simulink model "CTC_3PPP"  (R2018b)
settings: Solver=ode3  StartTime=0.0  StopTime=7  FixedStep=1e-3  RelTol=1e-3  EnableMultiTasking=on
undefined symbols (not defined in the file or in its folder): X, Y, Z
libraries: sm_lib x53, nesl_utility x13, simulink x2
(part 1 of 2)
settings Model: Creator=ledan  LastModifiedBy=oattao
settings DataIOCC: LimitDataPoints=on  SaveFormat=Array
settings OptimizationCC: LifeSpan=inf
settings DebuggingCC: UnderspecifiedInitializationDetection=Classic  MergeDetectMultiDrivingBlocksExec=none  SolverPrmCheckMsg=warning  StateNameClashWarn=warning  SFUnexpectedBacktrackingDiag=warning  SFNoUnconditionalDefaultTransitionDiag=warning  SFExecutionAtInitializationDiag=none
settings HardwareCC: ProdBitPerPointer=32  ProdBitPerSizeT=32  ProdBitPerPtrDiffT=32  ProdLargestAtomicFloat=None  ProdIntDivRoundTo=Undefined  ProdEndianess=Unspecified  ProdWordSize=32  ProdHWDeviceType=32-bit Generic
settings ModelReferenceCC: PropagateSignalLabelsOutOfModel=off
settings SFSimCC: SimUseLocalCustomCode=off
settings RTWCC: RTWUseLocalCustomCode=off
settings CodeAppCC: StateflowObjectComments=on
settings GRTTargetCC: TargetLangStandard=C89/C90 (ANSI)  GeneratePreprocessorConditionals=Disable all
settings ConfigComp: CovMetricSettings=dw  CovHtmlReporting=on  CovSaveCumulativeToWorkspaceVar=on  CovSaveSingleToWorkspaceVar=on  CovExternalEMLEnable=off
settings SimscapeCC: SimscapeNormalizeSystem=off
settings ConfigurationSet: Description=SimMechanics 2G

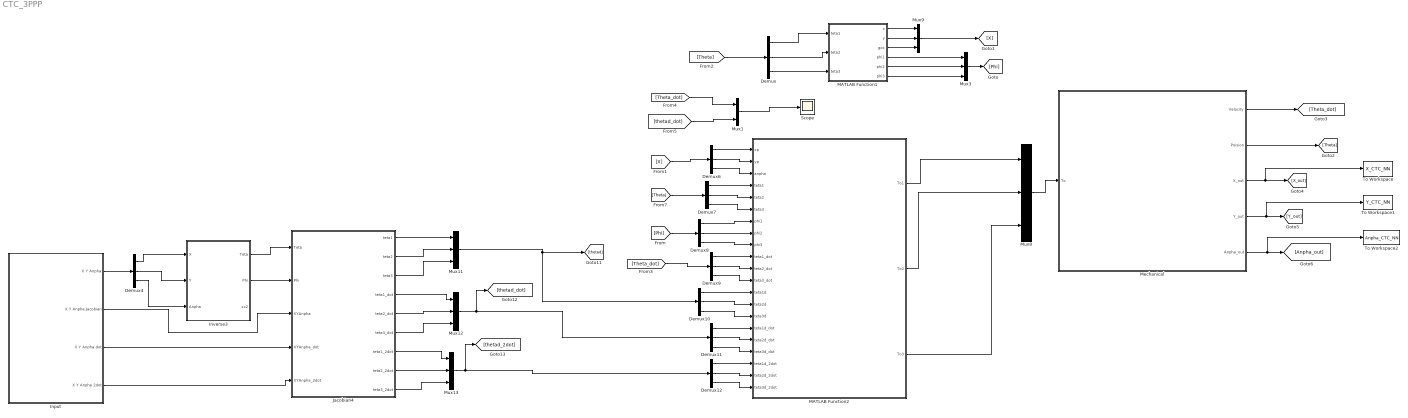
== system CTC_3PPP ==
  Demux{,4,6..12} (9 alike) : Demux  Outputs=3
  Input : Subsystem
  Inverse3 : Subsystem
  Jacobian4 : Subsystem
  MATLAB Function1 : MATLAB Function  TreatAsAtomicUnit=on
  MATLAB Function2 : MATLAB Function  TreatAsAtomicUnit=on
  Mechanical : Subsystem
      mask Display: image('RRR.jpg')
  Mux1 : Mux  Inputs=2
  Mux{3,8..9,11..13} (6 alike) : Mux  Inputs=3
  Scope : Scope
  To Workspace : ToWorkspace  VariableName=X_CTC_NN  SampleTime=-1
  To Workspace1 : ToWorkspace  VariableName=Y_CTC_NN  SampleTime=-1
  To Workspace2 : ToWorkspace  VariableName=Anpha_CTC_NN  SampleTime=-1
  wires:
  Demux/1 -> MATLAB Function1/1(teta1)
  Demux/2 -> MATLAB Function1/2(teta2)
  Demux/3 -> MATLAB Function1/3(teta3)
  MATLAB Function1/4(phi1) -> Mux3/1
  MATLAB Function1/5(phi2) -> Mux3/2
  MATLAB Function1/6(phi3) -> Mux3/3
  Mux12/1 -> [thetad_dot], Demux11/1
  Mux13/1 -> [thetad_2dot], Demux12/1
  Mechanical/1(Velocity) -> [Theta_dot]
  Mechanical/2(Poision) -> [Theta]
  Demux6/1 -> MATLAB Function2/1(xp)
  Demux6/2 -> MATLAB Function2/2(yp)
  Demux6/3 -> MATLAB Function2/3(anpha)
  Demux7/1 -> MATLAB Function2/4(teta1)
  Demux7/2 -> MATLAB Function2/5(teta2)
  Demux7/3 -> MATLAB Function2/6(teta3)
  Demux8/1 -> MATLAB Function2/7(phi1)
  Demux8/2 -> MATLAB Function2/8(phi2)
  Demux8/3 -> MATLAB Function2/9(phi3)
  Demux9/1 -> MATLAB Function2/10(teta1_dot)
  Demux9/2 -> MATLAB Function2/11(teta2_dot)
  Demux9/3 -> MATLAB Function2/12(teta3_dot)
  Demux10/1 -> MATLAB Function2/13(teta1d)
  Demux10/2 -> MATLAB Function2/14(teta2d)
  Demux10/3 -> MATLAB Function2/15(teta3d)
  Demux11/1 -> MATLAB Function2/16(teta1d_dot)
  Demux11/2 -> MATLAB Function2/17(teta2d_dot)
  Demux11/3 -> MATLAB Function2/18(teta3d_dot)
  Demux12/1 -> MATLAB Function2/19(teta1d_2dot)
  Demux12/2 -> MATLAB Function2/20(teta2d_2dot)
  Demux12/3 -> MATLAB Function2/21(teta3d_2dot)
  MATLAB Function1/1(x) -> Mux9/1
  MATLAB Function1/2(y) -> Mux9/2
  MATLAB Function1/3(goc) -> Mux9/3
  Mux3/1 -> [Phi]
  [Phi] -> Demux8/1
  Mux9/1 -> [X]
  [X] -> Demux6/1
  [Theta] -> Demux/1
  [Theta_dot] -> Demux9/1
  [Theta] -> Demux7/1
  Mechanical/3(X_out) -> [X_out], To Workspace/1
  Mechanical/4(Y_out) -> To Workspace1/1, [Y_out]
  Mechanical/5(Anpha_out) -> To Workspace2/1, [Anpha_out]
  Mux11/1 -> [thetad], Demux10/1
  Input/1(X Y Anpha) -> Demux4/1
  Input/2(X Y Anpha Jacobian) -> Jacobian4/3(XYAnpha)
  Input/3(X Y Anpha dot) -> Jacobian4/4(XYAnpha_dot)
  Input/4(X Y Anpha 2dot) -> Jacobian4/5(XYAnpha_2dot)
  Demux4/1 -> Inverse3/1(X)
  Demux4/2 -> Inverse3/2(Y)
  Demux4/3 -> Inverse3/3(Anpha)
  Inverse3/1(Teta) -> Jacobian4/1(Teta)
  Inverse3/2(Phi) -> Jacobian4/2(Phi)
  Jacobian4/1(teta1) -> Mux11/1
  Jacobian4/2(teta2) -> Mux11/2
  Jacobian4/3(teta3) -> Mux11/3
  Jacobian4/4(teta1_dot) -> Mux12/1
  Jacobian4/5(teta2_dot) -> Mux12/2
  Jacobian4/6(teta3_dot) -> Mux12/3
  Jacobian4/7(teta1_2dot) -> Mux13/1
  Jacobian4/8(teta2_2dot) -> Mux13/2
  Jacobian4/9(teta3_2dot) -> Mux13/3
  Mux8/1 -> Mechanical/1(To)
  [Theta_dot] -> Mux1/1
  [thetad_dot] -> Mux1/2
  Mux1/1 -> Scope/1
  MATLAB Function2/1(To1) -> Mux8/1
  MATLAB Function2/2(To2) -> Mux8/2
  MATLAB Function2/3(To3) -> Mux8/3

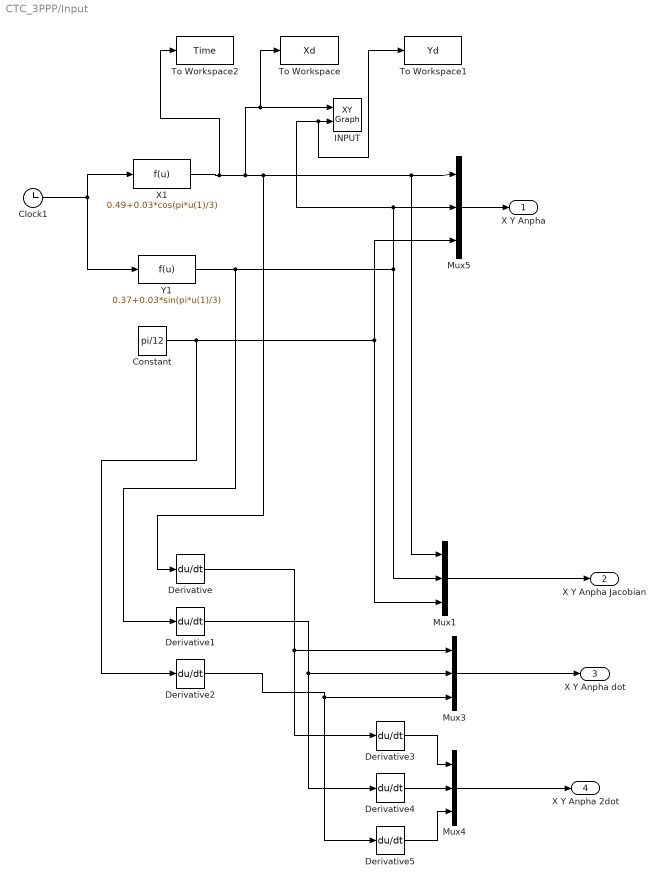
== system CTC_3PPP/Input ==
  Clock1 : Clock
  Constant : Constant  Value=pi/12
  Derivative{,1..5} (6 alike) : Derivative
  INPUT : simulink/Sinks/XY Graph  xmin=0.4  xmax=0.6  ymin=0.3  ymax=0.5  st=-1
  Mux{1,3..5} (4 alike) : Mux  Inputs=3
  To Workspace : ToWorkspace  VariableName=Xd  SampleTime=-1
  To Workspace1 : ToWorkspace  VariableName=Yd  SampleTime=-1
  To Workspace2 : ToWorkspace  VariableName=Time  SaveFormat=Timeseries  SampleTime=-1
  X1 : Fcn  Expr=0.49+0.03*cos(pi*u(1)/3)
  Y1 : Fcn  Expr=0.37+0.03*sin(pi*u(1)/3)
  X Y Anpha : Outport
  X Y Anpha Jacobian : Outport  Port=2
  X Y Anpha dot : Outport  Port=3
  X Y Anpha 2dot : Outport  Port=4
  wires:
  Derivative1/1 -> Mux3/2, Derivative4/1
  Derivative2/1 -> Mux3/3, Derivative5/1
  X1/1 -> To Workspace2/1, Derivative/1, Mux5/1, Mux1/1, To Workspace/1, INPUT/1
  Derivative3/1 -> Mux4/1
  Clock1/1 -> Y1/1, X1/1
  Y1/1 -> Derivative1/1, Mux1/2, To Workspace1/1, INPUT/2, Mux5/2
  Derivative/1 -> Mux3/1, Derivative3/1
  Derivative5/1 -> Mux4/3
  Derivative4/1 -> Mux4/2
  Constant/1 -> Mux1/3, Mux5/3, Derivative2/1
  Mux3/1 -> X Y Anpha dot/1
  Mux4/1 -> X Y Anpha 2dot/1
  Mux1/1 -> X Y Anpha Jacobian/1
  Mux5/1 -> X Y Anpha/1

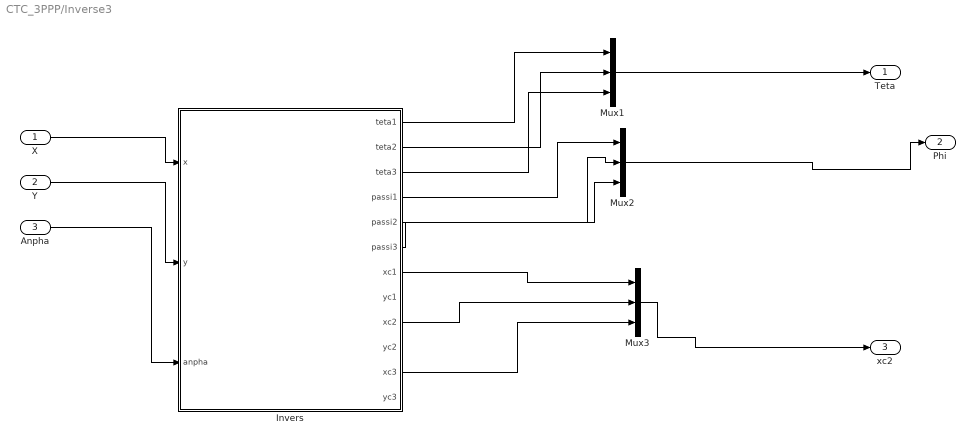
== system CTC_3PPP/Inverse3 ==
  X : Inport
  Y : Inport  Port=2
  Anpha : Inport  Port=3
  Invers : MATLAB Function  TreatAsAtomicUnit=on
  Mux1 : Mux  Inputs=3
  Mux2 : Mux  Inputs=3
  Mux3 : Mux  Inputs=3
  Teta : Outport
  Phi : Outport  Port=2
  xc2 : Outport  Port=3
  wires:
  Mux1/1 -> Teta/1
  Invers/6(passi3) -> Mux2/3
  Invers/3(teta3) -> Mux1/3
  Invers/1(teta1) -> Mux1/1
  Invers/2(teta2) -> Mux1/2
  Invers/4(passi1) -> Mux2/1
  Y/1 -> Invers/2(y)
  Anpha/1 -> Invers/3(anpha)
  X/1 -> Invers/1(x)
  Mux2/1 -> Phi/1
  Invers/5(passi2) -> Mux2/2
  Invers/7(xc1) -> Mux3/1
  Invers/11(xc3) -> Mux3/3
  Mux3/1 -> xc2/1
  Invers/9(xc2) -> Mux3/2

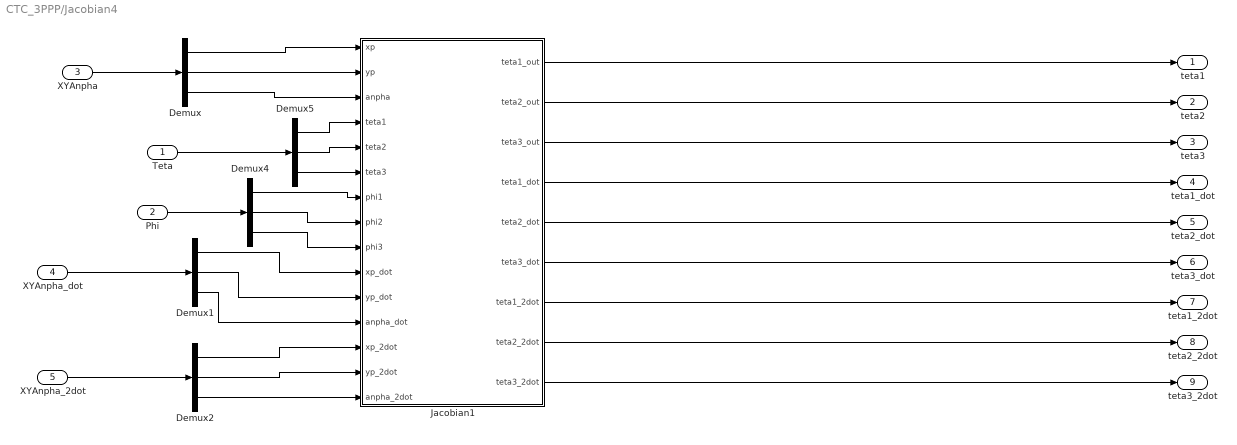
== system CTC_3PPP/Jacobian4 ==
  Teta : Inport
  Phi : Inport  Port=2
  XYAnpha : Inport  Port=3
  XYAnpha_dot : Inport  Port=4
  XYAnpha_2dot : Inport  Port=5
  Demux{,1..2,4..5} (5 alike) : Demux  Outputs=3
  Jacobian1 : MATLAB Function  TreatAsAtomicUnit=on
  teta1 : Outport
  teta2 : Outport  Port=2
  teta3 : Outport  Port=3
  teta1_dot : Outport  Port=4
  teta2_dot : Outport  Port=5
  teta3_dot : Outport  Port=6
  teta1_2dot : Outport  Port=7
  teta2_2dot : Outport  Port=8
  teta3_2dot : Outport  Port=9
  wires:
  XYAnpha_2dot/1 -> Demux2/1
  XYAnpha_dot/1 -> Demux1/1
  XYAnpha/1 -> Demux/1
  Demux/1 -> Jacobian1/1(xp)
  Demux4/2 -> Jacobian1/8(phi2)
  Demux2/3 -> Jacobian1/15(anpha_2dot)
  Demux2/1 -> Jacobian1/13(xp_2dot)
  Demux5/2 -> Jacobian1/5(teta2)
  Demux1/1 -> Jacobian1/10(xp_dot)
  Demux5/1 -> Jacobian1/4(teta1)
  Demux/2 -> Jacobian1/2(yp)
  Demux1/2 -> Jacobian1/11(yp_dot)
  Demux1/3 -> Jacobian1/12(anpha_dot)
  Demux2/2 -> Jacobian1/14(yp_2dot)
  Jacobian1/1(teta1_out) -> teta1/1
  Phi/1 -> Demux4/1
  Demux4/1 -> Jacobian1/7(phi1)
  Demux/3 -> Jacobian1/3(anpha)
  Demux5/3 -> Jacobian1/6(teta3)
  Teta/1 -> Demux5/1
  Jacobian1/3(teta3_out) -> teta3/1
  Demux4/3 -> Jacobian1/9(phi3)
  Jacobian1/2(teta2_out) -> teta2/1
  Jacobian1/6(teta3_dot) -> teta3_dot/1
  Jacobian1/4(teta1_dot) -> teta1_dot/1
  Jacobian1/5(teta2_dot) -> teta2_dot/1
  Jacobian1/7(teta1_2dot) -> teta1_2dot/1
  Jacobian1/8(teta2_2dot) -> teta2_2dot/1
  Jacobian1/9(teta3_2dot) -> teta3_2dot/1

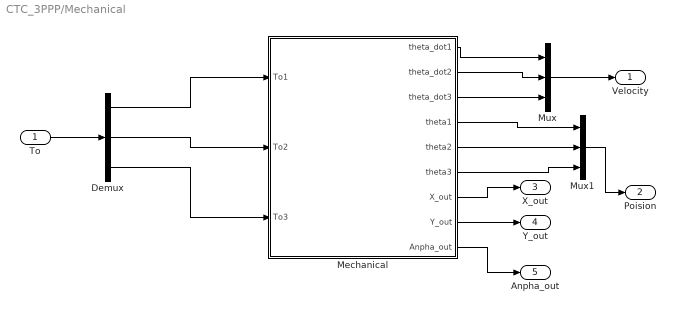
== system CTC_3PPP/Mechanical ==
  To : Inport
  Demux : Demux  Outputs=3
  Mechanical : Subsystem
  Mux : Mux  Inputs=3
  Mux1 : Mux  Inputs=3
  Velocity : Outport
  Poision : Outport  Port=2
  X_out : Outport  Port=3
  Y_out : Outport  Port=4
  Anpha_out : Outport  Port=5
  wires:
  Mechanical/3(theta_dot3) -> Mux/3
  Mechanical/1(theta_dot1) -> Mux/1
  Mechanical/5(theta2) -> Mux1/2
  Mechanical/6(theta3) -> Mux1/3
  Mechanical/4(theta1) -> Mux1/1
  Mux1/1 -> Poision/1
  Mechanical/2(theta_dot2) -> Mux/2
  To/1 -> Demux/1
  Mux/1 -> Velocity/1
  Demux/2 -> Mechanical/2(To2)
  Demux/3 -> Mechanical/3(To3)
  Mechanical/7(X_out) -> X_out/1
  Mechanical/8(Y_out) -> Y_out/1
  Mechanical/9(Anpha_out) -> Anpha_out/1
  Demux/1 -> Mechanical/1(To1)

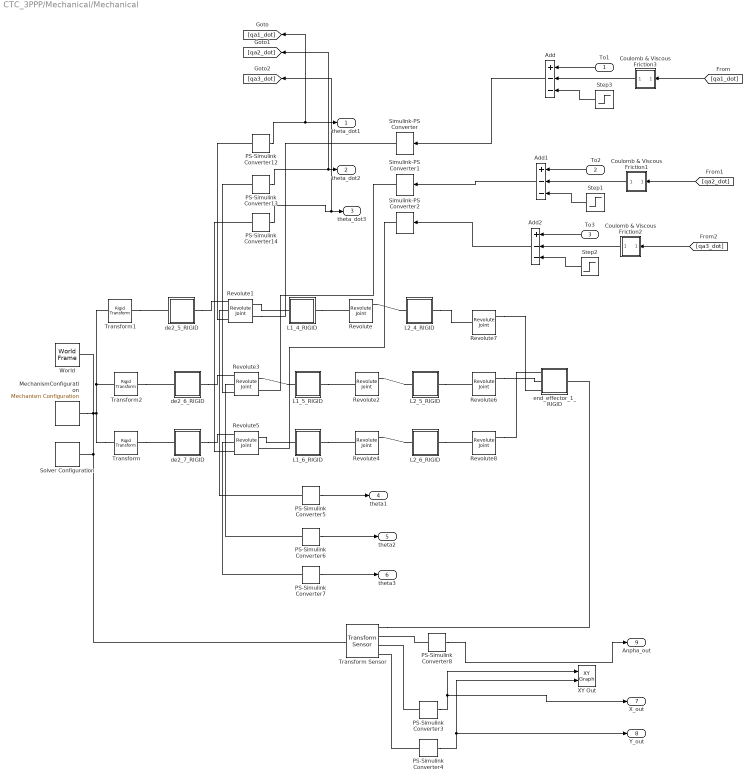
== system CTC_3PPP/Mechanical/Mechanical ==
  To1 : Inport
  To2 : Inport  Port=2
  To3 : Inport  Port=3
  Add : Sum  Inputs=+--
  Add1 : Sum  Inputs=+--
  Add2 : Sum  Inputs=+--
  Coulomb & Viscous Friction1 : Subsystem  AncestorBlock=simulink/Discontinuities/Coulomb & Viscous Friction  mask(Coulombic and Viscous Friction){offset=0.4, gain=0.5}
      mask prompts: offset "Coulomb friction value (Offset):"; gain "Coefficient of viscous friction (Gain):"
      mask help:
      | A discontinuity offset at zero models coulomb friction.  Linear gain models viscous friction.
      | y = sign(x) * (Gain * abs(x) + Offset)
      mask init:
      | dblOffset = double(offset(1));
      | dblGain = double(gain(1));
      | x=max(dblOffset,dblGain+dblOffset);
      mask Help:
      | This block has a discontinuity
      | at zero and a linear gain afterward.
      | y= sign(x)*(Gain*abs(x)+Offset)
      mask Display:
      | plot([-1 0 0 1],[-dblGain-dblOffset, -dblOffset, ...
      |     dblOffset, dblGain+dblOffset],...
      |     [-1 1],[0 0],[0 0],[-x,x])
  Coulomb & Viscous Friction2 : Subsystem  AncestorBlock=simulink/Discontinuities/Coulomb & Viscous Friction  mask(Coulombic and Viscous Friction){offset=0.4, gain=0.5}
      mask prompts: offset "Coulomb friction value (Offset):"; gain "Coefficient of viscous friction (Gain):"
      mask help:
      | A discontinuity offset at zero models coulomb friction.  Linear gain models viscous friction.
      | y = sign(x) * (Gain * abs(x) + Offset)
      mask init:
      | dblOffset = double(offset(1));
      | dblGain = double(gain(1));
      | x=max(dblOffset,dblGain+dblOffset);
      mask Help:
      | This block has a discontinuity
      | at zero and a linear gain afterward.
      | y= sign(x)*(Gain*abs(x)+Offset)
      mask Display:
      | plot([-1 0 0 1],[-dblGain-dblOffset, -dblOffset, ...
      |     dblOffset, dblGain+dblOffset],...
      |     [-1 1],[0 0],[0 0],[-x,x])
  Coulomb & Viscous Friction3 : Subsystem  AncestorBlock=simulink/Discontinuities/Coulomb & Viscous Friction  mask(Coulombic and Viscous Friction){offset=0.4, gain=0.5}
      mask prompts: offset "Coulomb friction value (Offset):"; gain "Coefficient of viscous friction (Gain):"
      mask help:
      | A discontinuity offset at zero models coulomb friction.  Linear gain models viscous friction.
      | y = sign(x) * (Gain * abs(x) + Offset)
      mask init:
      | dblOffset = double(offset(1));
      | dblGain = double(gain(1));
      | x=max(dblOffset,dblGain+dblOffset);
      mask Help:
      | This block has a discontinuity
      | at zero and a linear gain afterward.
      | y= sign(x)*(Gain*abs(x)+Offset)
      mask Display:
      | plot([-1 0 0 1],[-dblGain-dblOffset, -dblOffset, ...
      |     dblOffset, dblGain+dblOffset],...
      |     [-1 1],[0 0],[0 0],[-x,x])
  L1_4_RIGID : Subsystem
  L1_5_RIGID : Subsystem
  L1_6_RIGID : Subsystem
  L2_4_RIGID : Subsystem
  L2_5_RIGID : Subsystem
  L2_6_RIGID : Subsystem
  MechanismConfiguration : sm_lib/Utilities/Mechanism Configuration  UniformGravity=Constant  GravityVector=[0 -9.81 0]  GravityUnits=m/s^2  LinearizationDelta=0.001
  PS-Simulink Converter{3..8,12..14} (9 alike) : nesl_utility/PS-Simulink Converter  PhysicalDomain=network_engine_domain  SubClassName=ps_output  LeftPortType=input  RightPortType=output  PseudoPeriodic=off  Frequencies=[]  Unit=1  AffineConversion=off
  Revolute : sm_lib/Joints/Revolute Joint  SenseConstraintForce=off  SenseConstraintForceX=off  SenseConstraintForceY=off  SenseConstraintForceZ=off  SenseConstraintTorque=off  SenseConstraintTorqueX=off  SenseConstraintTorqueY=off  SenseConstraintTorqueZ=off  SenseTotalForce=off  SenseTotalForceX=off  SenseTotalForceY=off  SenseTotalForceZ=off  SenseTotalTorque=off  SenseTotalTorqueX=off  SenseTotalTorqueY=off  SenseTotalTorqueZ=off  CompositeWrenchDir=FollowerOnBase  CompositeWrenchFrame=BaseFrame  EquilibriumPosition=0  EquilibriumPositionUnits=rad  SpringStiffness=0  SpringStiffnessUnits=m*N/rad  DampingCoefficient=0  DampingCoefficientUnits=m*s*N/rad  TorqueActuationMode=NoTorque  MotionActuationMode=ComputedMotion  SensePosition=on  SenseVelocity=off  SenseAcceleration=off  SenseTorqueForce=off  PositionTargetSpecify=on  PositionTargetPriority=Low  PositionTargetValue=-2.4388  PositionTargetValueUnits=rad  VelocityTargetSpecify=off  VelocityTargetPriority=High  VelocityTargetValue=0  VelocityTargetValueUnits=deg/s
  Revolute1 : sm_lib/Joints/Revolute Joint  SenseConstraintForce=off  SenseConstraintForceX=off  SenseConstraintForceY=off  SenseConstraintForceZ=off  SenseConstraintTorque=off  SenseConstraintTorqueX=off  SenseConstraintTorqueY=off  SenseConstraintTorqueZ=off  SenseTotalForce=off  SenseTotalForceX=off  SenseTotalForceY=off  SenseTotalForceZ=off  SenseTotalTorque=off  SenseTotalTorqueX=off  SenseTotalTorqueY=off  SenseTotalTorqueZ=off  CompositeWrenchDir=FollowerOnBase  CompositeWrenchFrame=BaseFrame  EquilibriumPosition=0  EquilibriumPositionUnits=rad  SpringStiffness=0  SpringStiffnessUnits=m*N/rad  DampingCoefficient=0  DampingCoefficientUnits=m*s*N/rad  TorqueActuationMode=InputTorque  MotionActuationMode=ComputedMotion  SensePosition=on  SenseVelocity=on  SenseAcceleration=off  SenseTorqueForce=off  PositionTargetSpecify=on  PositionTargetPriority=Low  PositionTargetValue=2.1636  PositionTargetValueUnits=rad  VelocityTargetSpecify=off  VelocityTargetPriority=High  VelocityTargetValue=0  VelocityTargetValueUnits=deg/s
  Revolute2 : sm_lib/Joints/Revolute Joint  SenseConstraintForce=off  SenseConstraintForceX=off  SenseConstraintForceY=off  SenseConstraintForceZ=off  SenseConstraintTorque=off  SenseConstraintTorqueX=off  SenseConstraintTorqueY=off  SenseConstraintTorqueZ=off  SenseTotalForce=off  SenseTotalForceX=off  SenseTotalForceY=off  SenseTotalForceZ=off  SenseTotalTorque=off  SenseTotalTorqueX=off  SenseTotalTorqueY=off  SenseTotalTorqueZ=off  CompositeWrenchDir=FollowerOnBase  CompositeWrenchFrame=BaseFrame  EquilibriumPosition=0  EquilibriumPositionUnits=rad  SpringStiffness=0  SpringStiffnessUnits=m*N/rad  DampingCoefficient=0  DampingCoefficientUnits=m*s*N/rad  TorqueActuationMode=NoTorque  MotionActuationMode=ComputedMotion  SensePosition=on  SenseVelocity=off  SenseAcceleration=off  SenseTorqueForce=off  PositionTargetSpecify=off  PositionTargetPriority=Low  PositionTargetValue=-2.1897  PositionTargetValueUnits=rad  VelocityTargetSpecify=off  VelocityTargetPriority=High  VelocityTargetValue=0  VelocityTargetValueUnits=deg/s
  Revolute3 : sm_lib/Joints/Revolute Joint  SenseConstraintForce=off  SenseConstraintForceX=off  SenseConstraintForceY=off  SenseConstraintForceZ=off  SenseConstraintTorque=off  SenseConstraintTorqueX=off  SenseConstraintTorqueY=off  SenseConstraintTorqueZ=off  SenseTotalForce=off  SenseTotalForceX=off  SenseTotalForceY=off  SenseTotalForceZ=off  SenseTotalTorque=off  SenseTotalTorqueX=off  SenseTotalTorqueY=off  SenseTotalTorqueZ=off  CompositeWrenchDir=FollowerOnBase  CompositeWrenchFrame=BaseFrame  EquilibriumPosition=0  EquilibriumPositionUnits=rad  SpringStiffness=0  SpringStiffnessUnits=m*N/rad  DampingCoefficient=0  DampingCoefficientUnits=m*s*N/rad  TorqueActuationMode=InputTorque  MotionActuationMode=ComputedMotion  SensePosition=on  SenseVelocity=on  SenseAcceleration=off  SenseTorqueForce=off  PositionTargetSpecify=on  PositionTargetPriority=Low  PositionTargetValue=4.02  PositionTargetValueUnits=rad  VelocityTargetSpecify=off  VelocityTargetPriority=High  VelocityTargetValue=0  VelocityTargetValueUnits=deg/s
  Revolute4 : sm_lib/Joints/Revolute Joint  SenseConstraintForce=off  SenseConstraintForceX=off  SenseConstraintForceY=off  SenseConstraintForceZ=off  SenseConstraintTorque=off  SenseConstraintTorqueX=off  SenseConstraintTorqueY=off  SenseConstraintTorqueZ=off  SenseTotalForce=off  SenseTotalForceX=off  SenseTotalForceY=off  SenseTotalForceZ=off  SenseTotalTorque=off  SenseTotalTorqueX=off  SenseTotalTorqueY=off  SenseTotalTorqueZ=off  CompositeWrenchDir=FollowerOnBase  CompositeWrenchFrame=BaseFrame  EquilibriumPosition=0  EquilibriumPositionUnits=rad  SpringStiffness=0  SpringStiffnessUnits=m*N/rad  DampingCoefficient=0  DampingCoefficientUnits=m*s*N/rad  TorqueActuationMode=NoTorque  MotionActuationMode=ComputedMotion  SensePosition=on  SenseVelocity=off  SenseAcceleration=off  SenseTorqueForce=off  PositionTargetSpecify=off  PositionTargetPriority=Low  PositionTargetValue=2.7158  PositionTargetValueUnits=rad  VelocityTargetSpecify=off  VelocityTargetPriority=High  VelocityTargetValue=0  VelocityTargetValueUnits=deg/s
  Revolute5 : sm_lib/Joints/Revolute Joint  SenseConstraintForce=off  SenseConstraintForceX=off  SenseConstraintForceY=off  SenseConstraintForceZ=off  SenseConstraintTorque=off  SenseConstraintTorqueX=off  SenseConstraintTorqueY=off  SenseConstraintTorqueZ=off  SenseTotalForce=off  SenseTotalForceX=off  SenseTotalForceY=off  SenseTotalForceZ=off  SenseTotalTorque=off  SenseTotalTorqueX=off  SenseTotalTorqueY=off  SenseTotalTorqueZ=off  CompositeWrenchDir=FollowerOnBase  CompositeWrenchFrame=BaseFrame  EquilibriumPosition=0  EquilibriumPositionUnits=rad  SpringStiffness=0  SpringStiffnessUnits=m*N/rad  DampingCoefficient=0  DampingCoefficientUnits=m*s*N/rad  TorqueActuationMode=InputTorque  MotionActuationMode=ComputedMotion  SensePosition=on  SenseVelocity=on  SenseAcceleration=off  SenseTorqueForce=off  PositionTargetSpecify=on  PositionTargetPriority=Low  PositionTargetValue=0.5  PositionTargetValueUnits=rad  VelocityTargetSpecify=off  VelocityTargetPriority=High  VelocityTargetValue=0  VelocityTargetValueUnits=deg/s
  Revolute6 : sm_lib/Joints/Revolute Joint  SenseConstraintForce=off  SenseConstraintForceX=off  SenseConstraintForceY=off  SenseConstraintForceZ=off  SenseConstraintTorque=off  SenseConstraintTorqueX=off  SenseConstraintTorqueY=off  SenseConstraintTorqueZ=off  SenseTotalForce=off  SenseTotalForceX=off  SenseTotalForceY=off  SenseTotalForceZ=off  SenseTotalTorque=off  SenseTotalTorqueX=off  SenseTotalTorqueY=off  SenseTotalTorqueZ=off  CompositeWrenchDir=FollowerOnBase  CompositeWrenchFrame=BaseFrame  EquilibriumPosition=0  EquilibriumPositionUnits=rad  SpringStiffness=0  SpringStiffnessUnits=m*N/rad  DampingCoefficient=0  DampingCoefficientUnits=m*s*N/rad  TorqueActuationMode=NoTorque  MotionActuationMode=ComputedMotion  SensePosition=on  SenseVelocity=off  SenseAcceleration=off  SenseTorqueForce=off  PositionTargetSpecify=off  PositionTargetPriority=Low  PositionTargetValue=0  PositionTargetValueUnits=rad  VelocityTargetSpecify=off  VelocityTargetPriority=High  VelocityTargetValue=0  VelocityTargetValueUnits=deg/s
  Revolute7 : sm_lib/Joints/Revolute Joint  SenseConstraintForce=off  SenseConstraintForceX=off  SenseConstraintForceY=off  SenseConstraintForceZ=off  SenseConstraintTorque=off  SenseConstraintTorqueX=off  SenseConstraintTorqueY=off  SenseConstraintTorqueZ=off  SenseTotalForce=off  SenseTotalForceX=off  SenseTotalForceY=off  SenseTotalForceZ=off  SenseTotalTorque=off  SenseTotalTorqueX=off  SenseTotalTorqueY=off  SenseTotalTorqueZ=off  CompositeWrenchDir=FollowerOnBase  CompositeWrenchFrame=BaseFrame  EquilibriumPosition=0  EquilibriumPositionUnits=rad  SpringStiffness=0  SpringStiffnessUnits=m*N/rad  DampingCoefficient=0  DampingCoefficientUnits=m*s*N/rad  TorqueActuationMode=NoTorque  MotionActuationMode=ComputedMotion  SensePosition=on  SenseVelocity=off  SenseAcceleration=off  SenseTorqueForce=off  PositionTargetSpecify=off  PositionTargetPriority=Low  PositionTargetValue=0  PositionTargetValueUnits=rad  VelocityTargetSpecify=off  VelocityTargetPriority=High  VelocityTargetValue=0  VelocityTargetValueUnits=deg/s
  Revolute8 : sm_lib/Joints/Revolute Joint  SenseConstraintForce=off  SenseConstraintForceX=off  SenseConstraintForceY=off  SenseConstraintForceZ=off  SenseConstraintTorque=off  SenseConstraintTorqueX=off  SenseConstraintTorqueY=off  SenseConstraintTorqueZ=off  SenseTotalForce=off  SenseTotalForceX=off  SenseTotalForceY=off  SenseTotalForceZ=off  SenseTotalTorque=off  SenseTotalTorqueX=off  SenseTotalTorqueY=off  SenseTotalTorqueZ=off  CompositeWrenchDir=FollowerOnBase  CompositeWrenchFrame=BaseFrame  EquilibriumPosition=0  EquilibriumPositionUnits=rad  SpringStiffness=0  SpringStiffnessUnits=m*N/rad  DampingCoefficient=0  DampingCoefficientUnits=m*s*N/rad  TorqueActuationMode=NoTorque  MotionActuationMode=ComputedMotion  SensePosition=on  SenseVelocity=off  SenseAcceleration=off  SenseTorqueForce=off  PositionTargetSpecify=off  PositionTargetPriority=Low  PositionTargetValue=0  PositionTargetValueUnits=rad  VelocityTargetSpecify=off  VelocityTargetPriority=High  VelocityTargetValue=0  VelocityTargetValueUnits=deg/s
  Simulink-PS Converter : nesl_utility/Simulink-PS Converter  PhysicalDomain=network_engine_domain  SubClassName=ps_input  LeftPortType=input  RightPortType=output  PseudoPeriodic=off  Frequencies=[]  NoiseDistribution=none  NoiseParameters=[]  Unit=1  AffineConversion=off  FilteringAndDerivatives=zero  SimscapeFilterOrder=1  InputFilterTimeConstant=0.001  UdotUserProvided=1
  Simulink-PS Converter1 : nesl_utility/Simulink-PS Converter  PhysicalDomain=network_engine_domain  SubClassName=ps_input  LeftPortType=input  RightPortType=output  PseudoPeriodic=off  Frequencies=[]  NoiseDistribution=none  NoiseParameters=[]  Unit=1  AffineConversion=off  FilteringAndDerivatives=zero  SimscapeFilterOrder=1  InputFilterTimeConstant=0.001  UdotUserProvided=1
  Simulink-PS Converter2 : nesl_utility/Simulink-PS Converter  PhysicalDomain=network_engine_domain  SubClassName=ps_input  LeftPortType=input  RightPortType=output  PseudoPeriodic=off  Frequencies=[]  NoiseDistribution=none  NoiseParameters=[]  Unit=1  AffineConversion=off  FilteringAndDerivatives=zero  SimscapeFilterOrder=1  InputFilterTimeConstant=0.001  UdotUserProvided=1
  Solver Configuration : nesl_utility/Solver Configuration  PhysicalDomain=network_engine_domain  SubClassName=solver  LeftPortType=input  RightPortType=generic  Tones=[]  Harmonics=[]  SimulateNoise=off  Profile=off  UseLocalSampling=off  EnableSwitchedLinearOptims=on  FrequencyDomain=off  UseCCode=off  RelTol=0.001  AbsTol=1e-06  MinStep=1e-09  ToWorkspace=off  RevertToSquareIcSolve=off  NumHomotopyIterations=100  PhasorMode=off  PhasorModeNumHarmonics=1  DoDC=off  ResidualTolerance=1e-09  UseLocalSolver=off  LocalSolverChoice=NE_BACKWARD_EULER_ADVANCER  LocalSolverSampleTime=0.001  DoFixedCost=off  MaxNonlinIter=3  MaxModeIter=2  LinearAlgebra=Sparse  EquationFormulation=NE_TIME_EF  DelaysMemoryBudget=1024  AutomaticFiltering=on  FilteringTimeConstant=0.001  PartitionStorageMethod=AS_NEEDED  PartitionMemoryBudget=1024
  Step1 : Step  Time=0.5  After=0.001  SampleTime=0
  Step2 : Step  Time=0.5  After=0.001  SampleTime=0
  Step3 : Step  Time=0.5  After=0.001  SampleTime=0
  Transform : sm_lib/Frames and Transforms/Rigid Transform  TranslationMethod=Cartesian  TranslationStandardOffset=0  TranslationLengthUnit=mm  TranslationStandardAxis=+Z  TranslationCartesianOffset=[500 0 866.02500000000009]  TranslationROffset=0  TranslationROffsetUnits=m  TranslationZOffset=0  TranslationZOffsetUnits=m  TranslationThetaOffset=0  TranslationThetaOffsetUnits=deg  RotationMethod=None  RotationAngleUnits=deg  RotationStandardAxis=+Z  RotationAngle=0  RotationArbitraryAxis=[0 0 1]  FollAlignAxisA=+X  BaseAlignAxisA=+Y  FollAlignAxisB=+Y  BaseAlignAxisB=+Z  RotationSequenceAxes=FollowerAxes  RotationSequence=XYX  RotationSequenceAngles=[0 0 0]  RotationSequenceAnglesUnits=deg  RotationMatrix=[1 0 0; 0 1 0; 0 0 1]
  Transform Sensor : sm_lib/Frames and Transforms/Transform Sensor  MeasurementFrame=World  SenseAngle=on  SenseAxis=off  SenseAngle1=off  SenseAngle2=off  SenseAngle3=off  SenseQ=off  SenseR=off  SenseOmegaX=off  SenseOmegaY=off  SenseOmegaZ=off  SenseOmega1=off  SenseOmega2=off  SenseOmega3=off  SenseQDot=off  SenseRDot=off  SenseAlphaX=off  SenseAlphaY=off  SenseAlphaZ=off  SenseAlpha1=off  SenseAlpha2=off  SenseAlpha3=off  SenseQDDot=off  SenseRDDot=off  SenseX=on  SenseY=off  SenseZ=on  SenseRad=off  SenseAzim=off  SenseDist=off  SenseInc=off  SenseXDot=off  SenseYDot=off  SenseZDot=off  SenseRadDot=off  SenseAzimDot=off  SenseDistDot=off  SenseIncDot=off  SenseXDDot=off  SenseYDDot=off  SenseZDDot=off  SenseRadDDot=off  SenseAzimDDot=off  SenseDistDDot=off  SenseIncDDot=off
  Transform1 : sm_lib/Frames and Transforms/Rigid Transform  TranslationMethod=None  TranslationStandardOffset=0  TranslationLengthUnit=m  TranslationStandardAxis=+Z  TranslationCartesianOffset=[0 0 0]  TranslationROffset=0  TranslationROffsetUnits=m  TranslationZOffset=0  TranslationZOffsetUnits=m  TranslationThetaOffset=0  TranslationThetaOffsetUnits=deg  RotationMethod=None  RotationAngleUnits=deg  RotationStandardAxis=+Z  RotationAngle=0  RotationArbitraryAxis=[0 0 1]  FollAlignAxisA=+X  BaseAlignAxisA=+Y  FollAlignAxisB=+Y  BaseAlignAxisB=+Z  RotationSequenceAxes=FollowerAxes  RotationSequence=XYX  RotationSequenceAngles=[0 0 0]  RotationSequenceAnglesUnits=deg  RotationMatrix=[1 0 0; 0 1 0; 0 0 1]
  Transform2 : sm_lib/Frames and Transforms/Rigid Transform  TranslationMethod=Cartesian  TranslationStandardOffset=0  TranslationLengthUnit=mm  TranslationStandardAxis=+Z  TranslationCartesianOffset=[1000 0 0]  TranslationROffset=0  TranslationROffsetUnits=m  TranslationZOffset=0  TranslationZOffsetUnits=m  TranslationThetaOffset=0  TranslationThetaOffsetUnits=deg  RotationMethod=None  RotationAngleUnits=deg  RotationStandardAxis=+Z  RotationAngle=0  RotationArbitraryAxis=[0 0 1]  FollAlignAxisA=+X  BaseAlignAxisA=+Y  FollAlignAxisB=+Y  BaseAlignAxisB=+Z  RotationSequenceAxes=FollowerAxes  RotationSequence=XYX  RotationSequenceAngles=[0 0 0]  RotationSequenceAnglesUnits=deg  RotationMatrix=[1 0 0; 0 1 0; 0 0 1]
  World : sm_lib/Frames and Transforms/World Frame
  XY Out : simulink/Sinks/XY Graph  xmin=0.4  xmax=0.6  ymin=0.3  ymax=0.5  st=-1
  de2_5_RIGID : Subsystem
  de2_6_RIGID : Subsystem
  de2_7_RIGID : Subsystem
  end_effector_1_RIGID : Subsystem
  theta_dot1 : Outport
  theta_dot2 : Outport  Port=2
  theta_dot3 : Outport  Port=3
  theta1 : Outport  Port=4
  theta2 : Outport  Port=5
  theta3 : Outport  Port=6
  X_out : Outport  Port=7
  Y_out : Outport  Port=8
  Anpha_out : Outport  Port=9
  wires:
  PS-Simulink Converter8/1 -> Anpha_out/1
  Add1/1 -> Simulink-PS Converter1/1
  Add/1 -> Simulink-PS Converter/1
  Add2/1 -> Simulink-PS Converter2/1
  PS-Simulink Converter3/1 -> X_out/1, XY Out/1
  PS-Simulink Converter4/1 -> Y_out/1, XY Out/2
  PS-Simulink Converter5/1 -> theta1/1
  PS-Simulink Converter7/1 -> theta3/1
  PS-Simulink Converter6/1 -> theta2/1
  PS-Simulink Converter14/1 -> [qa3_dot], theta_dot3/1
  PS-Simulink Converter13/1 -> [qa2_dot], theta_dot2/1
  Coulomb & Viscous Friction3/1(Out1) -> Add/2
  Step3/1 -> Add/3
  [qa1_dot] -> Coulomb & Viscous Friction3/1(In1)
  To1/1 -> Add/1
  PS-Simulink Converter12/1 -> [qa1_dot], theta_dot1/1
  Coulomb & Viscous Friction1/1(Out1) -> Add1/2
  Step1/1 -> Add1/3
  [qa2_dot] -> Coulomb & Viscous Friction1/1(In1)
  To2/1 -> Add1/1
  Coulomb & Viscous Friction2/1(Out1) -> Add2/2
  Step2/1 -> Add2/3
  [qa3_dot] -> Coulomb & Viscous Friction2/1(In1)
  To3/1 -> Add2/1
  connections:
  de2_6_RIGID/RConn1 -- Revolute3/RConn1
  PS-Simulink Converter3/LConn1 -- Transform Sensor/RConn3
  Revolute5/LConn1 -- L1_6_RIGID/LConn1
  de2_7_RIGID/RConn1 -- Revolute5/RConn1
  L2_4_RIGID/RConn1 -- Revolute7/LConn1
  PS-Simulink Converter4/LConn1 -- Transform Sensor/RConn4
  PS-Simulink Converter8/LConn1 -- Transform Sensor/RConn2
  Simulink-PS Converter1/RConn1 -- Revolute3/LConn2
  Revolute1/LConn2 -- Simulink-PS Converter/RConn1
  L2_5_RIGID/RConn1 -- Revolute6/LConn1
  Simulink-PS Converter2/RConn1 -- Revolute5/LConn2
  Transform/LConn1 -- Transform1/LConn1 -- Transform2/LConn1 -- MechanismConfiguration/RConn1 -- Transform Sensor/LConn1 -- Solver Configuration/RConn1 -- World/RConn1
  L1_4_RIGID/RConn1 -- Revolute/LConn1
  L2_6_RIGID/LConn1 -- Revolute4/RConn1
  Revolute1/RConn2 -- PS-Simulink Converter5/LConn1
  L2_4_RIGID/LConn1 -- Revolute/RConn1
  PS-Simulink Converter7/LConn1 -- Revolute5/RConn2
  PS-Simulink Converter6/LConn1 -- Revolute3/RConn2
  de2_5_RIGID/RConn1 -- Revolute1/RConn1
  Revolute1/LConn1 -- L1_4_RIGID/LConn1
  Transform1/RConn1 -- de2_5_RIGID/LConn1
  L1_5_RIGID/LConn1 -- Revolute3/LConn1
  Transform2/RConn1 -- de2_6_RIGID/LConn1
  L1_6_RIGID/RConn1 -- Revolute4/LConn1
  L2_5_RIGID/LConn1 -- Revolute2/RConn1
  Transform/RConn1 -- de2_7_RIGID/LConn1
  L1_5_RIGID/RConn1 -- Revolute2/LConn1
  Transform Sensor/RConn1 -- end_effector_1_RIGID/RConn1
  PS-Simulink Converter14/LConn1 -- Revolute5/RConn3
  PS-Simulink Converter13/LConn1 -- Revolute3/RConn3
  PS-Simulink Converter12/LConn1 -- Revolute1/RConn3
  L2_6_RIGID/RConn1 -- Revolute8/LConn1
  Revolute7/RConn1 -- end_effector_1_RIGID/LConn3
  Revolute6/RConn1 -- end_effector_1_RIGID/LConn2
  Revolute8/RConn1 -- end_effector_1_RIGID/LConn1

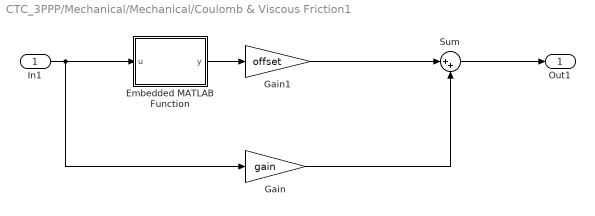
== system CTC_3PPP/Mechanical/Mechanical/Coulomb & Viscous Friction1 ==
  In1 : Inport
  Embedded MATLAB Function : MATLAB Function  TreatAsAtomicUnit=on
  Gain : Gain  DisableCoverage=on  Gain=gain  SaturateOnIntegerOverflow=on  OutDataTypeStr=Inherit: Same as input
  Gain1 : Gain  DisableCoverage=on  Gain=offset  OutDataTypeStr=Inherit: Inherit via back propagation  SaturateOnIntegerOverflow=on
  Sum : Sum  Inputs=|++  SaturateOnIntegerOverflow=on  InputSameDT=on  OutDataTypeStr=Inherit: Same as first input
  Out1 : Outport
  wires:
  Embedded MATLAB Function/1(y) -> Gain1/1
  In1/1 -> Embedded MATLAB Function/1(u), Gain/1
  Gain1/1 -> Sum/1
  Sum/1 -> Out1/1
  Gain/1 -> Sum/2

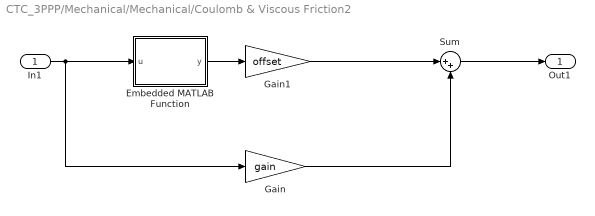
== system CTC_3PPP/Mechanical/Mechanical/Coulomb & Viscous Friction2 ==
  In1 : Inport
  Embedded MATLAB Function : MATLAB Function  TreatAsAtomicUnit=on
  Gain : Gain  DisableCoverage=on  Gain=gain  SaturateOnIntegerOverflow=on  OutDataTypeStr=Inherit: Same as input
  Gain1 : Gain  DisableCoverage=on  Gain=offset  OutDataTypeStr=Inherit: Inherit via back propagation  SaturateOnIntegerOverflow=on
  Sum : Sum  Inputs=|++  SaturateOnIntegerOverflow=on  InputSameDT=on  OutDataTypeStr=Inherit: Same as first input
  Out1 : Outport
  wires:
  Gain/1 -> Sum/2
  Sum/1 -> Out1/1
  Gain1/1 -> Sum/1
  In1/1 -> Gain/1, Embedded MATLAB Function/1(u)
  Embedded MATLAB Function/1(y) -> Gain1/1

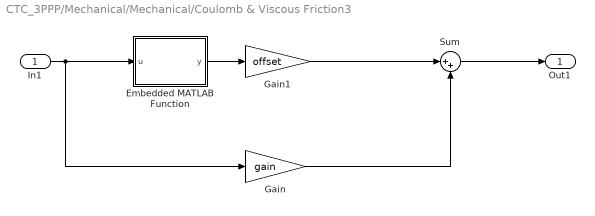
== system CTC_3PPP/Mechanical/Mechanical/Coulomb & Viscous Friction3 ==
  In1 : Inport
  Embedded MATLAB Function : MATLAB Function  TreatAsAtomicUnit=on
  Gain : Gain  DisableCoverage=on  Gain=gain  SaturateOnIntegerOverflow=on  OutDataTypeStr=Inherit: Same as input
  Gain1 : Gain  DisableCoverage=on  Gain=offset  OutDataTypeStr=Inherit: Inherit via back propagation  SaturateOnIntegerOverflow=on
  Sum : Sum  Inputs=|++  SaturateOnIntegerOverflow=on  InputSameDT=on  OutDataTypeStr=Inherit: Same as first input
  Out1 : Outport
  wires:
  Gain/1 -> Sum/2
  Sum/1 -> Out1/1
  Gain1/1 -> Sum/1
  In1/1 -> Gain/1, Embedded MATLAB Function/1(u)
  Embedded MATLAB Function/1(y) -> Gain1/1

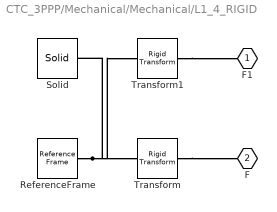
== system CTC_3PPP/Mechanical/Mechanical/L1_4_RIGID ==
  ReferenceFrame : sm_lib/Frames and Transforms/Reference Frame
  Solid : sm_lib/Body Elements/Solid  InertiaType=Custom  Mass=5.11836  MassUnits=kg  CenterOfMass=[-200 -10 0]  CenterOfMassUnits=mm  MomentsOfInertia=[2874.1399999999999 91391.700000000012 88858.699999999997]  MomentsOfInertiaUnits=kg*mm^2  ProductsOfInertia=[0 0 0]  ProductsOfInertiaUnits=kg*mm^2  BasedOnType=Density  Density=1000  DensityUnits=kg/(m^3)  DoExposeReferenceFrame=on  SerializedFrames=<Frames/>  GraphicType=FromGeometry  MarkerShape=Sphere  MarkerSize=10  MarkerSizeUnits=m  GraphicVisPropType=SimpleVisualProperties  GraphicDiffuseColor=[0.909804 0.443137 0.0313725]  GraphicSpecularColor=[0.5 0.5 0.5 1.0]  GraphicAmbientColor=[0.15 0.15 0.15 1.0]  GraphicEmissiveColor=[0.0 0.0 0.0 1.0]  GraphicShininess=75  GraphicOpacity=1  GeometryShape=FromFile  RectangleSize=[1 1]  RectangleSizeUnits=m  BrickDimensions=[1 1 1]  BrickDimensionUnits=m  CylinderRadius=1  CylinderRadiusUnits=m  CylinderLength=1  CylinderLengthUnits=m  SphereRadius=1  SphereRadiusUnits=m  EllipsoidRadii=[1 1 1]  EllipsoidRadiiUnits=m  ExtrusionCrossSection=[1 1; -1 1; -1 -1; 1 -1]  ExtrusionCrossSectionUnits=m  ExtrusionLength=1  ExtrusionLengthUnits=m  PolygonNumSides=3  PolygonOuterRadius=1  PolygonOuterRadiusUnits=m  ExtGeomFileType=STL  ExtGeomFileName=L1_Default_sldprt.STL  ExtGeomFileUnits=mm  RevolutionCrossSection=[1 1; 1 -1; 2 -1; 2 1]  RevolutionCrossSectionUnits=m  RevolutionExtent=Full  RevolutionAngle=180  RevolutionAngleUnits=deg
  Transform : sm_lib/Frames and Transforms/Rigid Transform  TranslationMethod=Cartesian  TranslationStandardOffset=0  TranslationLengthUnit=mm  TranslationStandardAxis=+Z  TranslationCartesianOffset=[0 0 0]  TranslationROffset=0  TranslationROffsetUnits=m  TranslationZOffset=0  TranslationZOffsetUnits=m  TranslationThetaOffset=0  TranslationThetaOffsetUnits=deg  RotationMethod=ArbitraryAxis  RotationAngleUnits=rad  RotationStandardAxis=+Z  RotationAngle=2.0943951023931953  RotationArbitraryAxis=[0.57735026918962584 -0.57735026918962584 0.57735026918962584]  FollAlignAxisA=+X  BaseAlignAxisA=+Y  FollAlignAxisB=+Y  BaseAlignAxisB=+Z  RotationSequenceAxes=FollowerAxes  RotationSequence=XYX  RotationSequenceAngles=[0 0 0]  RotationSequenceAnglesUnits=deg  RotationMatrix=[1 0 0; 0 1 0; 0 0 1]
  Transform1 : sm_lib/Frames and Transforms/Rigid Transform  TranslationMethod=Cartesian  TranslationStandardOffset=0  TranslationLengthUnit=mm  TranslationStandardAxis=+Z  TranslationCartesianOffset=[-399.99989135950761 -23.000000000002721 -0.000618050709306317]  TranslationROffset=0  TranslationROffsetUnits=m  TranslationZOffset=0  TranslationZOffsetUnits=m  TranslationThetaOffset=0  TranslationThetaOffsetUnits=deg  RotationMethod=ArbitraryAxis  RotationAngleUnits=rad  RotationStandardAxis=+Z  RotationAngle=2.0943951023931953  RotationArbitraryAxis=[-0.57735026918962584 -0.57735026918962584 -0.57735026918962584]  FollAlignAxisA=+X  BaseAlignAxisA=+Y  FollAlignAxisB=+Y  BaseAlignAxisB=+Z  RotationSequenceAxes=FollowerAxes  RotationSequence=XYX  RotationSequenceAngles=[0 0 0]  RotationSequenceAnglesUnits=deg  RotationMatrix=[1 0 0; 0 1 0; 0 0 1]
  F1 : PMIOPort  Side=Left
  F : PMIOPort  Port=2  Side=Right
  connections:
  Solid/RConn1 -- ReferenceFrame/RConn1 -- Transform/LConn1 -- Transform1/LConn1
  Transform/RConn1 -- F/RConn1
  Transform1/RConn1 -- F1/RConn1

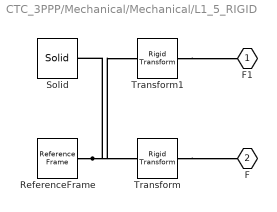
== system CTC_3PPP/Mechanical/Mechanical/L1_5_RIGID ==
  ReferenceFrame : sm_lib/Frames and Transforms/Reference Frame
  Solid : sm_lib/Body Elements/Solid  InertiaType=Custom  Mass=5.11836  MassUnits=kg  CenterOfMass=[-200 -10 0]  CenterOfMassUnits=mm  MomentsOfInertia=[2874.1399999999999 91391.700000000012 88858.699999999997]  MomentsOfInertiaUnits=kg*mm^2  ProductsOfInertia=[0 0 0]  ProductsOfInertiaUnits=kg*mm^2  BasedOnType=Density  Density=1000  DensityUnits=kg/(m^3)  DoExposeReferenceFrame=on  SerializedFrames=<Frames/>  GraphicType=FromGeometry  MarkerShape=Sphere  MarkerSize=10  MarkerSizeUnits=m  GraphicVisPropType=SimpleVisualProperties  GraphicDiffuseColor=[0.909804 0.443137 0.0313725]  GraphicSpecularColor=[0.5 0.5 0.5 1.0]  GraphicAmbientColor=[0.15 0.15 0.15 1.0]  GraphicEmissiveColor=[0.0 0.0 0.0 1.0]  GraphicShininess=75  GraphicOpacity=1  GeometryShape=FromFile  RectangleSize=[1 1]  RectangleSizeUnits=m  BrickDimensions=[1 1 1]  BrickDimensionUnits=m  CylinderRadius=1  CylinderRadiusUnits=m  CylinderLength=1  CylinderLengthUnits=m  SphereRadius=1  SphereRadiusUnits=m  EllipsoidRadii=[1 1 1]  EllipsoidRadiiUnits=m  ExtrusionCrossSection=[1 1; -1 1; -1 -1; 1 -1]  ExtrusionCrossSectionUnits=m  ExtrusionLength=1  ExtrusionLengthUnits=m  PolygonNumSides=3  PolygonOuterRadius=1  PolygonOuterRadiusUnits=m  ExtGeomFileType=STL  ExtGeomFileName=L1_Default_sldprt.STL  ExtGeomFileUnits=mm  RevolutionCrossSection=[1 1; 1 -1; 2 -1; 2 1]  RevolutionCrossSectionUnits=m  RevolutionExtent=Full  RevolutionAngle=180  RevolutionAngleUnits=deg
  Transform : sm_lib/Frames and Transforms/Rigid Transform  TranslationMethod=Cartesian  TranslationStandardOffset=0  TranslationLengthUnit=mm  TranslationStandardAxis=+Z  TranslationCartesianOffset=[0 0 0]  TranslationROffset=0  TranslationROffsetUnits=m  TranslationZOffset=0  TranslationZOffsetUnits=m  TranslationThetaOffset=0  TranslationThetaOffsetUnits=deg  RotationMethod=ArbitraryAxis  RotationAngleUnits=rad  RotationStandardAxis=+Z  RotationAngle=2.0943951023931953  RotationArbitraryAxis=[0.57735026918962584 -0.57735026918962584 0.57735026918962584]  FollAlignAxisA=+X  BaseAlignAxisA=+Y  FollAlignAxisB=+Y  BaseAlignAxisB=+Z  RotationSequenceAxes=FollowerAxes  RotationSequence=XYX  RotationSequenceAngles=[0 0 0]  RotationSequenceAnglesUnits=deg  RotationMatrix=[1 0 0; 0 1 0; 0 0 1]
  Transform1 : sm_lib/Frames and Transforms/Rigid Transform  TranslationMethod=Cartesian  TranslationStandardOffset=0  TranslationLengthUnit=mm  TranslationStandardAxis=+Z  TranslationCartesianOffset=[-400.00008703101673 -22.999999999997851 0.00042320257364281133]  TranslationROffset=0  TranslationROffsetUnits=m  TranslationZOffset=0  TranslationZOffsetUnits=m  TranslationThetaOffset=0  TranslationThetaOffsetUnits=deg  RotationMethod=ArbitraryAxis  RotationAngleUnits=rad  RotationStandardAxis=+Z  RotationAngle=2.0943951023931957  RotationArbitraryAxis=[-0.57735026918962584 -0.57735026918962573 -0.57735026918962573]  FollAlignAxisA=+X  BaseAlignAxisA=+Y  FollAlignAxisB=+Y  BaseAlignAxisB=+Z  RotationSequenceAxes=FollowerAxes  RotationSequence=XYX  RotationSequenceAngles=[0 0 0]  RotationSequenceAnglesUnits=deg  RotationMatrix=[1 0 0; 0 1 0; 0 0 1]
  F1 : PMIOPort  Side=Left
  F : PMIOPort  Port=2  Side=Right
  connections:
  Solid/RConn1 -- ReferenceFrame/RConn1 -- Transform/LConn1 -- Transform1/LConn1
  Transform/RConn1 -- F/RConn1
  Transform1/RConn1 -- F1/RConn1

== system CTC_3PPP/Mechanical/Mechanical/L1_6_RIGID ==
  ReferenceFrame : sm_lib/Frames and Transforms/Reference Frame
  Solid : sm_lib/Body Elements/Solid  InertiaType=Custom  Mass=5.11836  MassUnits=kg  CenterOfMass=[-200 -10 0]  CenterOfMassUnits=mm  MomentsOfInertia=[2874.1399999999999 91391.700000000012 88858.699999999997]  MomentsOfInertiaUnits=kg*mm^2  ProductsOfInertia=[0 0 0]  ProductsOfInertiaUnits=kg*mm^2  BasedOnType=Density  Density=1000  DensityUnits=kg/(m^3)  DoExposeReferenceFrame=on  SerializedFrames=<Frames/>  GraphicType=FromGeometry  MarkerShape=Sphere  MarkerSize=10  MarkerSizeUnits=m  GraphicVisPropType=SimpleVisualProperties  GraphicDiffuseColor=[0.909804 0.443137 0.0313725]  GraphicSpecularColor=[0.5 0.5 0.5 1.0]  GraphicAmbientColor=[0.15 0.15 0.15 1.0]  GraphicEmissiveColor=[0.0 0.0 0.0 1.0]  GraphicShininess=75  GraphicOpacity=1  GeometryShape=FromFile  RectangleSize=[1 1]  RectangleSizeUnits=m  BrickDimensions=[1 1 1]  BrickDimensionUnits=m  CylinderRadius=1  CylinderRadiusUnits=m  CylinderLength=1  CylinderLengthUnits=m  SphereRadius=1  SphereRadiusUnits=m  EllipsoidRadii=[1 1 1]  EllipsoidRadiiUnits=m  ExtrusionCrossSection=[1 1; -1 1; -1 -1; 1 -1]  ExtrusionCrossSectionUnits=m  ExtrusionLength=1  ExtrusionLengthUnits=m  PolygonNumSides=3  PolygonOuterRadius=1  PolygonOuterRadiusUnits=m  ExtGeomFileType=STL  ExtGeomFileName=L1_Default_sldprt.STL  ExtGeomFileUnits=mm  RevolutionCrossSection=[1 1; 1 -1; 2 -1; 2 1]  RevolutionCrossSectionUnits=m  RevolutionExtent=Full  RevolutionAngle=180  RevolutionAngleUnits=deg
  Transform : sm_lib/Frames and Transforms/Rigid Transform  TranslationMethod=Cartesian  TranslationStandardOffset=0  TranslationLengthUnit=mm  TranslationStandardAxis=+Z  TranslationCartesianOffset=[0 0 0]  TranslationROffset=0  TranslationROffsetUnits=m  TranslationZOffset=0  TranslationZOffsetUnits=m  TranslationThetaOffset=0  TranslationThetaOffsetUnits=deg  RotationMethod=ArbitraryAxis  RotationAngleUnits=rad  RotationStandardAxis=+Z  RotationAngle=2.0943951023931953  RotationArbitraryAxis=[0.57735026918962584 -0.57735026918962584 0.57735026918962584]  FollAlignAxisA=+X  BaseAlignAxisA=+Y  FollAlignAxisB=+Y  BaseAlignAxisB=+Z  RotationSequenceAxes=FollowerAxes  RotationSequence=XYX  RotationSequenceAngles=[0 0 0]  RotationSequenceAnglesUnits=deg  RotationMatrix=[1 0 0; 0 1 0; 0 0 1]
  Transform1 : sm_lib/Frames and Transforms/Rigid Transform  TranslationMethod=Cartesian  TranslationStandardOffset=0  TranslationLengthUnit=mm  TranslationStandardAxis=+Z  TranslationCartesianOffset=[-400.00274016823732 -23.000000000002053 -0.002627075484042507]  TranslationROffset=0  TranslationROffsetUnits=m  TranslationZOffset=0  TranslationZOffsetUnits=m  TranslationThetaOffset=0  TranslationThetaOffsetUnits=deg  RotationMethod=ArbitraryAxis  RotationAngleUnits=rad  RotationStandardAxis=+Z  RotationAngle=2.0943951023931957  RotationArbitraryAxis=[-0.57735026918962584 -0.57735026918962584 -0.57735026918962562]  FollAlignAxisA=+X  BaseAlignAxisA=+Y  FollAlignAxisB=+Y  BaseAlignAxisB=+Z  RotationSequenceAxes=FollowerAxes  RotationSequence=XYX  RotationSequenceAngles=[0 0 0]  RotationSequenceAnglesUnits=deg  RotationMatrix=[1 0 0; 0 1 0; 0 0 1]
  F1 : PMIOPort  Side=Left
  F : PMIOPort  Port=2  Side=Right
  connections:
  Solid/RConn1 -- ReferenceFrame/RConn1 -- Transform/LConn1 -- Transform1/LConn1
  Transform/RConn1 -- F/RConn1
  Transform1/RConn1 -- F1/RConn1

== system CTC_3PPP/Mechanical/Mechanical/L2_4_RIGID ==
  ReferenceFrame : sm_lib/Frames and Transforms/Reference Frame
  Solid : sm_lib/Body Elements/Solid  InertiaType=Custom  Mass=7.3903600000000003  MassUnits=kg  CenterOfMass=[-300 -10 0]  CenterOfMassUnits=mm  MomentsOfInertia=[4161.6100000000006 267638 263969]  MomentsOfInertiaUnits=kg*mm^2  ProductsOfInertia=[0 0 0]  ProductsOfInertiaUnits=kg*mm^2  BasedOnType=Density  Density=1000  DensityUnits=kg/(m^3)  DoExposeReferenceFrame=on  SerializedFrames=<Frames/>  GraphicType=FromGeometry  MarkerShape=Sphere  MarkerSize=10  MarkerSizeUnits=m  GraphicVisPropType=SimpleVisualProperties  GraphicDiffuseColor=[0.909804 0.443137 0.0313725]  GraphicSpecularColor=[0.5 0.5 0.5 1.0]  GraphicAmbientColor=[0.15 0.15 0.15 1.0]  GraphicEmissiveColor=[0.0 0.0 0.0 1.0]  GraphicShininess=75  GraphicOpacity=1  GeometryShape=FromFile  RectangleSize=[1 1]  RectangleSizeUnits=m  BrickDimensions=[1 1 1]  BrickDimensionUnits=m  CylinderRadius=1  CylinderRadiusUnits=m  CylinderLength=1  CylinderLengthUnits=m  SphereRadius=1  SphereRadiusUnits=m  EllipsoidRadii=[1 1 1]  EllipsoidRadiiUnits=m  ExtrusionCrossSection=[1 1; -1 1; -1 -1; 1 -1]  ExtrusionCrossSectionUnits=m  ExtrusionLength=1  ExtrusionLengthUnits=m  PolygonNumSides=3  PolygonOuterRadius=1  PolygonOuterRadiusUnits=m  ExtGeomFileType=STL  ExtGeomFileName=L2_Default_sldprt.STL  ExtGeomFileUnits=mm  RevolutionCrossSection=[1 1; 1 -1; 2 -1; 2 1]  RevolutionCrossSectionUnits=m  RevolutionExtent=Full  RevolutionAngle=180  RevolutionAngleUnits=deg
  Transform : sm_lib/Frames and Transforms/Rigid Transform  TranslationMethod=Cartesian  TranslationStandardOffset=0  TranslationLengthUnit=mm  TranslationStandardAxis=+Z  TranslationCartesianOffset=[-600.00074171908818 20.000000000000878 -0.00073761782886094807]  TranslationROffset=0  TranslationROffsetUnits=m  TranslationZOffset=0  TranslationZOffsetUnits=m  TranslationThetaOffset=0  TranslationThetaOffsetUnits=deg  RotationMethod=ArbitraryAxis  RotationAngleUnits=rad  RotationStandardAxis=+Z  RotationAngle=2.0943951023931962  RotationArbitraryAxis=[0.57735026918962584 -0.57735026918962584 0.5773502691896254]  FollAlignAxisA=+X  BaseAlignAxisA=+Y  FollAlignAxisB=+Y  BaseAlignAxisB=+Z  RotationSequenceAxes=FollowerAxes  RotationSequence=XYX  RotationSequenceAngles=[0 0 0]  RotationSequenceAnglesUnits=deg  RotationMatrix=[1 0 0; 0 1 0; 0 0 1]
  Transform1 : sm_lib/Frames and Transforms/Rigid Transform  TranslationMethod=Cartesian  TranslationStandardOffset=0  TranslationLengthUnit=mm  TranslationStandardAxis=+Z  TranslationCartesianOffset=[0 0 0]  TranslationROffset=0  TranslationROffsetUnits=m  TranslationZOffset=0  TranslationZOffsetUnits=m  TranslationThetaOffset=0  TranslationThetaOffsetUnits=deg  RotationMethod=ArbitraryAxis  RotationAngleUnits=rad  RotationStandardAxis=+Z  RotationAngle=2.0943951023931953  RotationArbitraryAxis=[0.57735026918962584 -0.57735026918962584 0.57735026918962584]  FollAlignAxisA=+X  BaseAlignAxisA=+Y  FollAlignAxisB=+Y  BaseAlignAxisB=+Z  RotationSequenceAxes=FollowerAxes  RotationSequence=XYX  RotationSequenceAngles=[0 0 0]  RotationSequenceAnglesUnits=deg  RotationMatrix=[1 0 0; 0 1 0; 0 0 1]
  F : PMIOPort  Side=Left
  F1 : PMIOPort  Port=2  Side=Right
  connections:
  Solid/RConn1 -- ReferenceFrame/RConn1 -- Transform/LConn1 -- Transform1/LConn1
  Transform/RConn1 -- F/RConn1
  Transform1/RConn1 -- F1/RConn1

== system CTC_3PPP/Mechanical/Mechanical/L2_5_RIGID ==
  ReferenceFrame : sm_lib/Frames and Transforms/Reference Frame
  Solid : sm_lib/Body Elements/Solid  InertiaType=Custom  Mass=7.3903600000000003  MassUnits=kg  CenterOfMass=[-300 -10 0]  CenterOfMassUnits=mm  MomentsOfInertia=[4161.6100000000006 267638 263969]  MomentsOfInertiaUnits=kg*mm^2  ProductsOfInertia=[0 0 0]  ProductsOfInertiaUnits=kg*mm^2  BasedOnType=Density  Density=1000  DensityUnits=kg/(m^3)  DoExposeReferenceFrame=on  SerializedFrames=<Frames/>  GraphicType=FromGeometry  MarkerShape=Sphere  MarkerSize=10  MarkerSizeUnits=m  GraphicVisPropType=SimpleVisualProperties  GraphicDiffuseColor=[0.909804 0.443137 0.0313725]  GraphicSpecularColor=[0.5 0.5 0.5 1.0]  GraphicAmbientColor=[0.15 0.15 0.15 1.0]  GraphicEmissiveColor=[0.0 0.0 0.0 1.0]  GraphicShininess=75  GraphicOpacity=1  GeometryShape=FromFile  RectangleSize=[1 1]  RectangleSizeUnits=m  BrickDimensions=[1 1 1]  BrickDimensionUnits=m  CylinderRadius=1  CylinderRadiusUnits=m  CylinderLength=1  CylinderLengthUnits=m  SphereRadius=1  SphereRadiusUnits=m  EllipsoidRadii=[1 1 1]  EllipsoidRadiiUnits=m  ExtrusionCrossSection=[1 1; -1 1; -1 -1; 1 -1]  ExtrusionCrossSectionUnits=m  ExtrusionLength=1  ExtrusionLengthUnits=m  PolygonNumSides=3  PolygonOuterRadius=1  PolygonOuterRadiusUnits=m  ExtGeomFileType=STL  ExtGeomFileName=L2_Default_sldprt.STL  ExtGeomFileUnits=mm  RevolutionCrossSection=[1 1; 1 -1; 2 -1; 2 1]  RevolutionCrossSectionUnits=m  RevolutionExtent=Full  RevolutionAngle=180  RevolutionAngleUnits=deg
  Transform : sm_lib/Frames and Transforms/Rigid Transform  TranslationMethod=Cartesian  TranslationStandardOffset=0  TranslationLengthUnit=mm  TranslationStandardAxis=+Z  TranslationCartesianOffset=[-600.00018421991467 19.999999999995772 0.0010338089975903131]  TranslationROffset=0  TranslationROffsetUnits=m  TranslationZOffset=0  TranslationZOffsetUnits=m  TranslationThetaOffset=0  TranslationThetaOffsetUnits=deg  RotationMethod=ArbitraryAxis  RotationAngleUnits=rad  RotationStandardAxis=+Z  RotationAngle=2.0943951023931953  RotationArbitraryAxis=[0.57735026918962584 -0.57735026918962584 0.57735026918962584]  FollAlignAxisA=+X  BaseAlignAxisA=+Y  FollAlignAxisB=+Y  BaseAlignAxisB=+Z  RotationSequenceAxes=FollowerAxes  RotationSequence=XYX  RotationSequenceAngles=[0 0 0]  RotationSequenceAnglesUnits=deg  RotationMatrix=[1 0 0; 0 1 0; 0 0 1]
  Transform1 : sm_lib/Frames and Transforms/Rigid Transform  TranslationMethod=Cartesian  TranslationStandardOffset=0  TranslationLengthUnit=mm  TranslationStandardAxis=+Z  TranslationCartesianOffset=[0 0 0]  TranslationROffset=0  TranslationROffsetUnits=m  TranslationZOffset=0  TranslationZOffsetUnits=m  TranslationThetaOffset=0  TranslationThetaOffsetUnits=deg  RotationMethod=ArbitraryAxis  RotationAngleUnits=rad  RotationStandardAxis=+Z  RotationAngle=2.0943951023931953  RotationArbitraryAxis=[0.57735026918962584 -0.57735026918962584 0.57735026918962584]  FollAlignAxisA=+X  BaseAlignAxisA=+Y  FollAlignAxisB=+Y  BaseAlignAxisB=+Z  RotationSequenceAxes=FollowerAxes  RotationSequence=XYX  RotationSequenceAngles=[0 0 0]  RotationSequenceAnglesUnits=deg  RotationMatrix=[1 0 0; 0 1 0; 0 0 1]
  F : PMIOPort  Side=Left
  F1 : PMIOPort  Port=2  Side=Right
  connections:
  Solid/RConn1 -- ReferenceFrame/RConn1 -- Transform/LConn1 -- Transform1/LConn1
  Transform/RConn1 -- F/RConn1
  Transform1/RConn1 -- F1/RConn1
